simulink model "Zimpedence_SZV2_3"  (R2017b)
settings: Solver=ode45  StartTime=0.0  StopTime=0.1  MaxStep=1e-6  RelTol=1e-3
InitFcn:
  | clear;
  | clc;
  | format long;
  | f = 85e3;
  | w = 2*pi*f;
  | 
  | Lp = 263e-6;
  | Cp = 1/(w^2*Lp);
  | 
  | M = 100e-6;
  | 
  | %%%%副边参数
  | Wz = 0.8*w;
  | %%%%%%%根据Z网络参数设计LsV2.1%%%%%%%
  | %Q = 5;
  | %RL= 20;
  | %Lz = RL*Q/w;
  | %Cz = w/RL/Wz^2/Q;
  | %Ls = 2*RL*Q/w/(w^2/Wz^2-1);
  | %CL = 2*w/RL/Wz^2/Q/(w^2/Wz^2-1);
  | 
  | %%%%%%%根据Z网络参数设计Ls V2.2%%%%%%%
  | %Lz = 387e-6;
  | %Cz = 1/Lz/Wz^2;
  | %Ls = 2*Lz/(w^2/Wz^2-1);
  | %CL = 2/Lz/Wz^2/(w^2/Wz^2-1);
  | 
  | %%%%%%根据增益和Ls求Lz V2 %%%%%%%%%
  | Ls =  258e-6;;
  | Lz = Ls*(w^2/Wz^2-1)/2;
  | Cz = 2/Ls/Wz^2/(w^2/Wz^2-1);
  | CL = 4/Ls/Wz^2/(w^2/Wz^2-1)^2;
libraries: powerlib x29, peRmsMeasurement x13, simulink x4, powerlib_meascontrol x4
settings Model: Creator=SuperWindows  LastModifiedBy=SuperWindows
settings DebuggingCC: UnconnectedInputMsg=none  UnconnectedOutputMsg=none  UnconnectedLineMsg=none

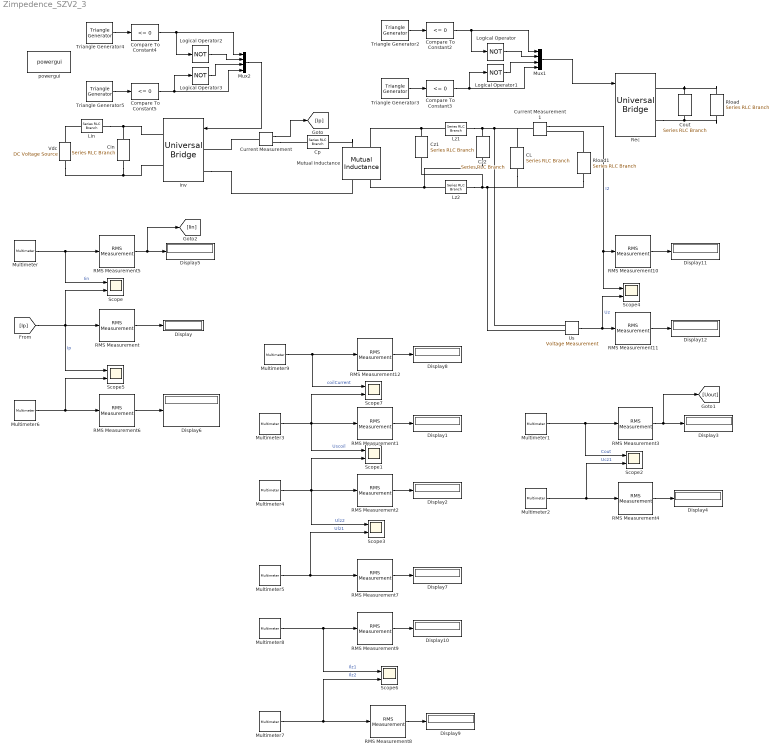
== system Zimpedence_SZV2_3 ==
  CL : powerlib/Elements/Series RLC Branch  LConnTagsString=__new0  RConnTagsString=__new0  BranchType=C  Resistance=1  Inductance=Lp  SetiL0=off  InitialCurrent=0  Capacitance=CL  Setx0=off  InitialVoltage=0  Measurements=Branch voltage and current
  Cin : powerlib/Elements/Series RLC Branch  LConnTagsString=__new0  RConnTagsString=__new0  BranchType=RC  Resistance=0.1  Inductance=Lz  SetiL0=off  InitialCurrent=0  Capacitance=10e-6  Setx0=off  InitialVoltage=0  Measurements=Branch voltage and current
  Compare To Constant{2..5} (4 alike) : simulink/Logic and Bit Operations/Compare To Constant  relop=<=  const=0  OutDataTypeStr=boolean
  Cout : powerlib/Elements/Series RLC Branch  LConnTagsString=__new0  RConnTagsString=__new0  BranchType=C  Resistance=1  Inductance=Lp  SetiL0=off  InitialCurrent=0  Capacitance=470e-6  Setx0=on  InitialVoltage=90  Measurements=Branch voltage and current
  Cp : powerlib/Elements/Series RLC Branch  LConnTagsString=__new0  RConnTagsString=__new0  BranchType=C  Resistance=0.5  Inductance=Lp  SetiL0=off  InitialCurrent=0  Capacitance=Cp  Setx0=off  InitialVoltage=0  Measurements=None
  Current Measurement : powerlib/Measurements/Current Measurement  PhasorSimulation=off  OutputType=Complex  PSBequivalent=0
  Current Measurement1 : powerlib/Measurements/Current Measurement  PhasorSimulation=off  OutputType=Complex  PSBequivalent=0
  Cz1 : powerlib/Elements/Series RLC Branch  LConnTagsString=__new0  RConnTagsString=__new0  BranchType=C  Resistance=1  Inductance=Lp  SetiL0=off  InitialCurrent=0  Capacitance=Cz  Setx0=off  InitialVoltage=0  Measurements=Branch voltage and current
  Cz2 : powerlib/Elements/Series RLC Branch  LConnTagsString=__new0  RConnTagsString=__new0  BranchType=C  Resistance=1  Inductance=Lp  SetiL0=off  InitialCurrent=0  Capacitance=Cz  Setx0=off  InitialVoltage=0  Measurements=Branch voltage and current
  Display{,1..12} (13 alike) : Display
  Lin : powerlib/Elements/Series RLC Branch  LConnTagsString=__new0  RConnTagsString=__new0  BranchType=L  Resistance=1  Inductance=10e-6  SetiL0=off  InitialCurrent=0  Capacitance=Cz  Setx0=off  InitialVoltage=0  Measurements=Branch voltage and current
  Logical Operator{,1..3} (4 alike) : Logic  Operator=NOT  AllPortsSameDT=off  OutDataTypeStr=boolean
  Lz1 : powerlib/Elements/Series RLC Branch  LConnTagsString=__new0  RConnTagsString=__new0  BranchType=L  Resistance=1  Inductance=Lz  SetiL0=off  InitialCurrent=0  Capacitance=Cz  Setx0=off  InitialVoltage=0  Measurements=Branch voltage and current
  Lz2 : powerlib/Elements/Series RLC Branch  LConnTagsString=__new0  RConnTagsString=__new0  BranchType=L  Resistance=1  Inductance=Lz  SetiL0=off  InitialCurrent=0  Capacitance=Cz  Setx0=off  InitialVoltage=0  Measurements=Branch voltage and current
  Multimeter : powerlib/Measurements/Multimeter  PhasorSimulation=off  OutputType=Complex  sel=29  L=44  Gain=1  yselected={'Ib: Lin'};  PSBOutputType=1  PSBequivalent=0  AxesSetting=[0,0.1,-100,100]  Display=0  SavedBlockNames=-11
  Multimeter1 : powerlib/Measurements/Multimeter  PhasorSimulation=off  OutputType=Complex  sel=8  L=44  Gain=1  yselected={'Ub: Rload'};  PSBOutputType=1  PSBequivalent=0  AxesSetting=[0,0.1,-100,100]  Display=0  SavedBlockNames=-11
  Multimeter2 : powerlib/Measurements/Multimeter  PhasorSimulation=off  OutputType=Complex  sel=3  L=44  Gain=1  yselected={'Ub: Cz1'};  PSBOutputType=1  PSBequivalent=0  AxesSetting=[0,0.1,-100,100]  Display=0  SavedBlockNames=-11
  Multimeter3 : powerlib/Measurements/Multimeter  PhasorSimulation=off  OutputType=Complex  sel=12  L=44  Gain=1  yselected={'Uw2: Mutual Inductance'};  PSBOutputType=1  PSBequivalent=0  AxesSetting=[0,0.1,-100,100]  Display=0  SavedBlockNames=-11
  Multimeter4 : powerlib/Measurements/Multimeter  PhasorSimulation=off  OutputType=Complex  sel=7  L=44  Gain=1  yselected={'Ub: Lz2'};  PSBOutputType=1  PSBequivalent=0  AxesSetting=[0,0.1,-100,100]  Display=0  SavedBlockNames=-11
  Multimeter5 : powerlib/Measurements/Multimeter  PhasorSimulation=off  OutputType=Complex  sel=6  L=44  Gain=1  yselected={'Ub: Lz1'};  PSBOutputType=1  PSBequivalent=0  AxesSetting=[0,0.1,-100,100]  Display=0  SavedBlockNames=-11
  Multimeter6 : powerlib/Measurements/Multimeter  PhasorSimulation=off  OutputType=Complex  sel=17  L=44  Gain=1  yselected={'Uab: inv'};  PSBOutputType=1  PSBequivalent=0  AxesSetting=[0,0.1,-100,100]  Display=0  SavedBlockNames=-11
  Multimeter7 : powerlib/Measurements/Multimeter  PhasorSimulation=off  OutputType=Complex  sel=31  L=44  Gain=1  yselected={'Ib: Lz2'};  PSBOutputType=1  PSBequivalent=0  AxesSetting=[0,0.1,-100,100]  Display=0  SavedBlockNames=-11
  Multimeter8 : powerlib/Measurements/Multimeter  PhasorSimulation=off  OutputType=Complex  sel=30  L=44  Gain=1  yselected={'Ib: Lz1'};  PSBOutputType=1  PSBequivalent=0  AxesSetting=[0,0.1,-100,100]  Display=0  SavedBlockNames=-11
  Multimeter9 : powerlib/Measurements/Multimeter  PhasorSimulation=off  OutputType=Complex  sel=36  L=44  Gain=1  yselected={'Iw2: Mutual Inductance'};  PSBOutputType=1  PSBequivalent=0  AxesSetting=[0,0.1,-100,100]  Display=0  SavedBlockNames=-11
  Mutual Inductance : powerlib/Elements/Mutual Inductance  LConnTagsString=a|b  RConnTagsString=A|B  TypeOfMutual=Two or three windings with equal mutual terms  NumberOfWindings=3  SelfImpedance1=[0.28 Lp]  SelfImpedance2=[0.3 Ls]  ThreeWindings=off  SelfImpedance3=[ 1.1 1.1e-03]  MutualImpedance=[0 M]  InductanceMatrix="[1.0 0.9  0.9 ;  0.9 1.0  0.9;  0.9 0.9 1.0 ] * 1e-3"  ResistanceMatrix="[1.0 0.9  0.9 ;  0.9 1.0  0.9;  0.9 0.9 1.0 ]"  Measurements=Winding voltages and currents
      settings: AttributesFormatString=\n  SourceProductName=Simscape Power Systems  SourceProductBaseCode=PS
  Mux1 : Mux
  Mux2 : Mux
  RMS Measurement{,1..4,7..12} (11 alike) : peRmsMeasurement/RMS Measurement  OverrideUsingVariant=Total  F=f  SpecifyHarmonics=off  K=[0 1 2]  Ts=0
  RMS Measurement5 : peRmsMeasurement/RMS Measurement  OverrideUsingVariant=Total  F=f/10  SpecifyHarmonics=off  K=[0 1 2]  Ts=0
  RMS Measurement6 : peRmsMeasurement/RMS Measurement  OverrideUsingVariant=Harmonic  F=f  SpecifyHarmonics=on  K=[0 1 2]  Ts=0
  Rec : powerlib/Power Electronics/Universal Bridge  Arms=2  SnubberResistance=1e5  SnubberCapacitance=inf  Device=MOSFET / Diodes  Ron=80e-3  Lon=0  ForwardVoltages="[  0  0  ]"  ForwardVoltage=0.45  GTOparameters=[ 10e-6 , 20e-6 ]  IGBTparameters=[ 1e-6 , 2e-6 ]  Measurements=All voltages and currents  Measurements_2=None  converterType=Rectifier
  Rload : powerlib/Elements/Series RLC Branch  LConnTagsString=__new0  RConnTagsString=__new0  BranchType=R  Resistance=6.17  Inductance=Lp  SetiL0=off  InitialCurrent=0  Capacitance=470e-6  Setx0=off  InitialVoltage=0  Measurements=Branch voltage and current
  Rload1 : powerlib/Elements/Series RLC Branch  LConnTagsString=__new0  RConnTagsString=__new0  BranchType=R  Resistance=5  Inductance=Lp  SetiL0=off  InitialCurrent=0  Capacitance=470e-6  Setx0=off  InitialVoltage=0  Measurements=Branch voltage and current
  Scope{,1..7} (8 alike) : Scope  NumInputPorts=2
  Triangle Generator2 : powerlib_meascontrol/Pulse & Signal Generators/Triangle Generator  Freq=f  Phase=270  Ts=0
  Triangle Generator3 : powerlib_meascontrol/Pulse & Signal Generators/Triangle Generator  Freq=f  Phase=270  Ts=0
  Triangle Generator4 : powerlib_meascontrol/Pulse & Signal Generators/Triangle Generator  Freq=f  Phase=0  Ts=0
  Triangle Generator5 : powerlib_meascontrol/Pulse & Signal Generators/Triangle Generator  Freq=f  Phase=0  Ts=0
  Us : powerlib/Measurements/Voltage Measurement  PhasorSimulation=off  OutputType=Complex  PSBequivalent=0
  Vdc : powerlib/Electrical Sources/DC Voltage Source  Amplitude=200  Measurements=None
  inv : powerlib/Power Electronics/Universal Bridge  Arms=2  SnubberResistance=1e5  SnubberCapacitance=inf  Device=MOSFET / Diodes  Ron=80e-3  Lon=0  ForwardVoltages="[  0  0  ]"  ForwardVoltage=0  GTOparameters=[ 10e-6 , 20e-6 ]  IGBTparameters=[ 1e-6 , 2e-6 ]  Measurements=All voltages and currents  Measurements_2=None  converterType=Rectifier
  powergui : powerlib/powergui  Priority=1  SimulationMode=Discrete  SampleTime=5e-8  frequency=60  Iterations=50  frequencyindice=0  Pbase=100e6  ErrMax=1e-4  UnitsV=kV  UnitsW=MW  buscounter=0  FunctionMessages=off  echomessages=off  EnableUseOfTLC=off  CurrentSourceSwitches=off  DisableSnubberDevices=off  DisableRonSwitches=off  DisableVfSwitches=off  DisplayEquations=off  SolverType=Tustin/Backward Euler (TBE)  Interpol=off  ExternalGateDelay=off  methode=off  Ts=100  x0status=blocks  SPID=on  SwTol=0  HookPort=off  RestoreLinks=warning  ResistiveCurrentMeasurement=off  Frange=[0:2:500]  Ylog=off  Xlog=on  ShowGrid=off  save=off  variable=ZData  structure=ULZ  ZoomFFT=off  StartTime=0.03135  cycles=30  DisplayStyle=2  fundamental=85e3  FreqAxis=off  MaxFrequency=100*85e3  frequencyindicesteady=1  RmsSteady=1  display=off
  wires:
  Compare To Constant2/1 -> Mux1/1, Logical Operator/1
  Triangle Generator3/1 -> Compare To Constant3/1
  Compare To Constant3/1 -> Mux1/4, Logical Operator1/1
  Triangle Generator2/1 -> Compare To Constant2/1
  Logical Operator1/1 -> Mux1/3
  Logical Operator/1 -> Mux1/2
  Logical Operator2/1 -> Mux2/2
  Logical Operator3/1 -> Mux2/3
  Triangle Generator4/1 -> Compare To Constant4/1
  Triangle Generator5/1 -> Compare To Constant5/1
  Compare To Constant5/1 -> Mux2/4, Logical Operator3/1
  Compare To Constant4/1 -> Mux2/1, Logical Operator2/1
  Mux2/1 -> inv/1
  Current Measurement/1 -> [Ip]
  [Ip] -> Scope/2, Scope5/1, RMS Measurement/1  "Ip"
  RMS Measurement1/1 -> Display1/1
  RMS Measurement2/1 -> Display2/1
  Multimeter4/1 -> Scope3/1, Scope1/2, RMS Measurement2/1  "Ulz2"
  RMS Measurement3/1 -> [Uout], Display3/1
  Multimeter1/1 -> Scope2/1, RMS Measurement3/1  "Cout"
  Multimeter2/1 -> RMS Measurement4/1, Scope2/2  "Ucz1"
  RMS Measurement4/1 -> Display4/1
  Multimeter3/1 -> Scope7/2, Scope1/1, RMS Measurement1/1  "Uscoil"
  Multimeter5/1 -> RMS Measurement7/1, Scope3/2  "Ulz1"
  Multimeter/1 -> Scope/1, RMS Measurement5/1  "Iin"
  RMS Measurement5/1 -> [Iin], Display5/1
  Current Measurement1/1 -> Scope4/1, RMS Measurement10/1  "I2"
  Us/1 -> Scope4/2, RMS Measurement11/1  "Uz"
  Multimeter6/1 -> Scope5/2, RMS Measurement6/1
  RMS Measurement7/1 -> Display7/1
  Mux1/1 -> Rec/1
  Multimeter7/1 -> RMS Measurement8/1, Scope6/2  "Ilz2"
  RMS Measurement8/1 -> Display9/1
  Multimeter8/1 -> RMS Measurement9/1, Scope6/1  "Ilz1"
  RMS Measurement9/1 -> Display10/1
  RMS Measurement10/1 -> Display11/1
  RMS Measurement11/1 -> Display12/1
  RMS Measurement12/1 -> Display8/1
  Multimeter9/1 -> Scope7/1, RMS Measurement12/1  "coilCurrent"
  RMS Measurement/1 -> Display/1
  RMS Measurement6/1 -> Display6/1
  connections:
  Mutual Inductance/LConn1 -- Cp/RConn1
  Vdc/LConn1 -- Cin/RConn1 -- inv/RConn2
  Lz1/LConn1 -- Mutual Inductance/LConn2 -- Cz1/LConn1
  Mutual Inductance/RConn2 -- Cz2/RConn1 -- Lz2/LConn1
  Lz2/RConn1 -- CL/RConn1 -- Rload1/RConn1 -- Us/LConn2 -- Cz1/RConn1
  Cout/LConn1 -- Rload/LConn1 -- Rec/RConn1
  Rload/RConn1 -- Rec/RConn2 -- Cout/RConn1
  Current Measurement/RConn1 -- Cp/LConn1
  Lin/LConn1 -- Vdc/RConn1
  Lin/RConn1 -- Cin/LConn1 -- inv/RConn1
  Current Measurement/LConn1 -- inv/LConn1
  inv/LConn2 -- Mutual Inductance/RConn1
  Lz1/RConn1 -- CL/LConn1 -- Current Measurement1/LConn1 -- Us/LConn1 -- Cz2/LConn1
  Rload1/LConn1 -- Current Measurement1/RConn1
